simulink model "EntrySend_2018a"  (R2018a)
settings: Solver=VariableStepAuto  StartTime=0.0  StopTime=10.0  RelTol=1e-3
settings Model: Creator=apple  LastModifiedBy=apple
settings DataIOCC: ReturnWorkspaceOutputs=on
settings SFSimCC: SimUseLocalCustomCode=on
settings RTWCC: RTWUseLocalCustomCode=on

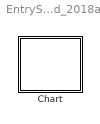
== system EntrySend_2018a ==
  Chart : Stateflow chart  TreatAsAtomicUnit=on

== stateflow chart EntrySend_2018a/Chart ==
  state A
    en:fprintf("Entry A");
    du:fprintf("During A");
    ex:fprintf("Exit A");
  state B
    en:fprintf("Entry B");send(F);
    du:fprintf("During B");
    ex:fprintf("Exit B");
  (default) -> A
  A -> B : E/{send(F);}
  B -> A : F
  events: E local FUNCTION_CALL_EVENT; F local FUNCTION_CALL_EVENT
